simulink model "adarbha_hw6_mdl"  (Simulink 7.7)
settings: Solver=ode1  StartTime=0.0  StopTime=max(time_s)  FixedStep=0.00001  RelTol=1e-5
InitFcn:
  | adarbha_hw6
values from neighbouring files (symbols this model uses):
  Area = 2.7    [adarbha_hw6.m]    (also in hw6.m; hw6_code.m)
  Cd = 0.44    [adarbha_hw6.m]    (also in hw6.m; hw6_code.m)
  density = 1.224    [adarbha_hw6.m]    (also in hw6.m; hw6_code.m)
  Q = 20    [adarbha_hw6.m]    (also in hw6_code.m)
  R_batt = 0.1    [adarbha_hw6.m]    (also in hw6_code.m)
  radius_wheel_m = 0.41    [adarbha_hw6.m]    (also in hw6.m; hw6_code.m)
  rpm = 1:5000    [adarbha_hw6.m]    (also in hw6.m; hw6_code.m)
  Time = xlsread('Malibu_20100929_highway_Baseline','A:A')    [adarbha_hw6.m]    (also in hw6.m; hw6_code.m)
  time_s = time_scale*100    [adarbha_hw6.m]    (also in hw6.m; hw6_code.m)
  V_o = 300    [adarbha_hw6.m]    (also in hw6_code.m)
  vel_m_s = M_number*3    [adarbha_hw6.m]    (also in hw6.m; hw6_code.m)
  Velocity_kph = xlsread('Malibu_20100929_highway_Baseline','B:B')    [adarbha_hw6.m]    (also in hw6.m; hw6_code.m)
  weight_N = 16000    [adarbha_hw6.m]    (also in hw6.m; hw6_code.m)
undefined symbols (not defined in the file or in its folder): torque
libraries: simulink x1
settings Model: Creator=Arjun  LastModifiedBy=Arjun
settings DataIOCC: SignalLogging=off

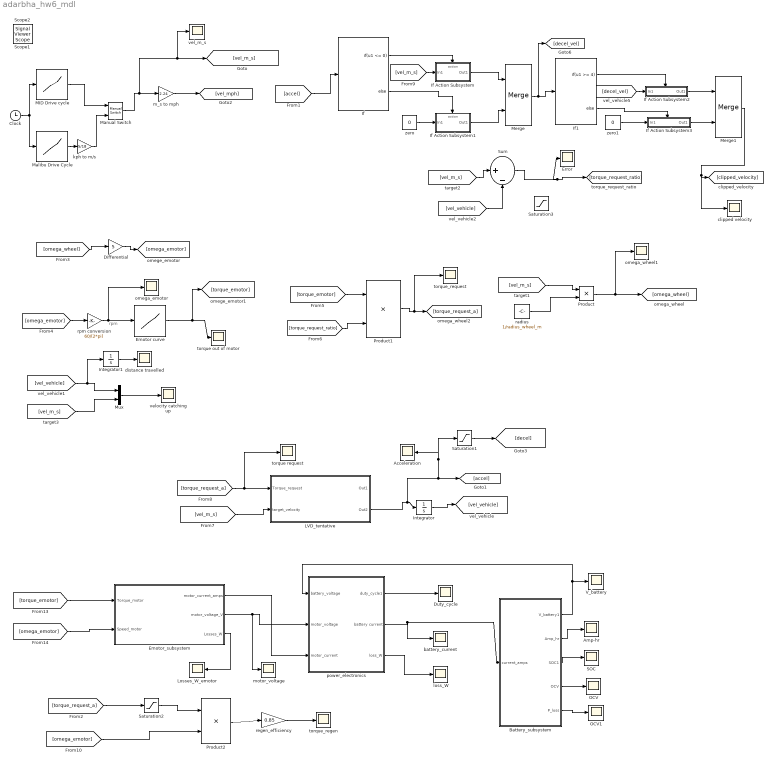
== system adarbha_hw6_mdl ==
  note: rpm
  Acceleration : Scope
      settings: SaveName=ScopeData11
  Amp-hr : Scope
      settings: SaveName=ScopeData23
  Battery_subsystem : Subsystem
      settings: MinAlgLoopOccurrences=on
  Clock : Clock
      settings: Decimation=10
  Differential : Gain  Gain=5
  Duty_cycle : Scope
      settings: SaveName=ScopeData22
  Emotor curve : Lookup_n-D  NumberOfTableDimensions=1  BreakpointsForDimension1=rpm  Table=torque  RndMeth=Simplest  InputSameDT=on
  Emotor_subsystem : Subsystem
  Error : Scope
      settings: SaveName=ScopeData17
  If : If  IfExpression=u1 <= 0
  If Action Subsystem : Subsystem  TreatAsAtomicUnit=on
  If Action Subsystem1 : Subsystem  TreatAsAtomicUnit=on
  If Action Subsystem2 : Subsystem  TreatAsAtomicUnit=on
  If Action Subsystem3 : Subsystem  TreatAsAtomicUnit=on
  If1 : If  IfExpression=u1 >= 4
  Integrator : Integrator
  Integrator1 : Integrator
  LVD_tentative : Subsystem
  Losses_W_emotor : Scope
      settings: SaveName=ScopeData19
  MID Drive cycle : Lookup_n-D  NumberOfTableDimensions=1  BreakpointsForDimension1=time_s  Table=vel_m_s  RndMeth=Simplest  InputSameDT=on
  Malibu Drive Cycle : Lookup_n-D  NumberOfTableDimensions=1  BreakpointsForDimension1=Time  Table=Velocity_kph  RndMeth=Simplest  InputSameDT=on
  Manual Switch : simulink/Signal Routing/Manual Switch  SystemSampleTime=-1  sw=1  action=0  varsize=off
  Merge : Merge
  Merge1 : Merge
  Mux : Mux  Inputs=2
  OCV : Scope
      settings: SaveName=ScopeData31
  OCV1 : Scope
      settings: SaveName=ScopeData33
  Product : Product  RndMeth=Zero
  Product1 : Product  RndMeth=Zero
  Product2 : Product  RndMeth=Zero
  SOC : Scope
      settings: SaveName=ScopeData28
  Saturation1 : Saturate  UpperLimit=0  LowerLimit=-100
  Saturation2 : Saturate  UpperLimit=0  LowerLimit=-Inf
  Saturation3 : Saturate  UpperLimit=1  LowerLimit=-1  ZeroCross=off
  Sum : Sum  Inputs=|+-
  V_battery : Scope
      settings: SaveName=ScopeData29
  battery_current : Scope
      settings: SaveName=ScopeData24
  clipped velocity : Scope
  distance travelled : Scope
      settings: SaveName=ScopeData25
  kph to m/s : Gain  Gain=5/18
  loss_W : Scope
      settings: SaveName=ScopeData20
  m_s to mph : Gain  Gain=2.24
  motor_voltage : Scope
      settings: SaveName=ScopeData26
  omega_emotor : Scope
      settings: SaveName=ScopeData7
  omega_wheel1 : Scope
      settings: SaveName=ScopeData4
  power_electronics : Subsystem
      settings: MinAlgLoopOccurrences=on
  radius : Constant  Value=1/radius_wheel_m
  regen_efficiency : Gain  Gain=0.85
  rpm conversion : Gain  Gain=60/(2*pi)
  torque out of motor : Scope
      settings: SaveName=ScopeData8
  torque request : Scope
      settings: SaveName=ScopeData12
  torque_regen : Scope
      settings: SaveName=ScopeData16
  torque_request : Scope
      settings: SaveName=ScopeData6
  vel_m_s : Scope
      settings: SaveName=ScopeData21
  velocity catching up : Scope
      settings: TimeRange=765.8724058416602  YMin=-1e+049  YMax=9.000000000000001e+049  SaveName=ScopeData18
  zero : Constant  Value=0
  zero1 : Constant  Value=0
  Scope1 : SignalViewerScope  IOType=viewer  NumInputPorts=5  RefreshTime=0.035000
  Scope2 : SignalViewerScope  IOType=viewer  RefreshTime=0.035000
  wires:
  m_s to mph/1 -> [vel_mph]
  Clock/1 -> MID Drive cycle/1, Malibu Drive Cycle/1
  [vel_m_s] -> Product/1
  Product/1 -> [omega_wheel], omega_wheel1/1
  radius/1 -> Product/2
  [torque_emotor] -> Product1/1
  [torque_request_ratio] -> Product1/2
  Product1/1 -> [torque_request_a], torque_request/1
  [omega_wheel] -> Differential/1
  Differential/1 -> [omega_emotor]
  [omega_emotor] -> rpm conversion/1
  rpm conversion/1 -> Emotor curve/1, omega_emotor/1
  Emotor curve/1 -> torque out of motor/1, [torque_emotor]
  [vel_m_s] -> LVD_tentative/2(target_velocity)
  [torque_request_a] -> LVD_tentative/1(Torque_request), torque request/1
  Integrator/1 -> [vel_vehicle]
  LVD_tentative/2(Out2) -> Integrator/1, [accel], Saturation1/1, Acceleration/1
  [vel_m_s] -> Sum/1
  [vel_vehicle] -> Sum/2
  [vel_m_s] -> Mux/2
  [vel_vehicle] -> Mux/1, Integrator1/1
  Mux/1 -> velocity catching up/1
  Sum/1 -> [torque_request_ratio], Error/1
  Saturation1/1 -> [decel]
  [accel] -> If/1
  If/1 -> If Action Subsystem/Action
  [vel_m_s] -> If Action Subsystem/1(In1)
  If/2 -> If Action Subsystem1/Action
  zero/1 -> If Action Subsystem1/1(In1)
  If Action Subsystem/1(Out1) -> Merge/1
  If Action Subsystem1/1(Out1) -> Merge/2
  Merge/1 -> If1/1, [decel_vel]
  If1/1 -> If Action Subsystem2/Action
  If1/2 -> If Action Subsystem3/Action
  [decel_vel] -> If Action Subsystem2/1(In1)
  zero1/1 -> If Action Subsystem3/1(In1)
  If Action Subsystem2/1(Out1) -> Merge1/1
  If Action Subsystem3/1(Out1) -> Merge1/2
  Merge1/1 -> clipped velocity/1, [clipped_velocity]
  MID Drive cycle/1 -> Manual Switch/1
  Manual Switch/1 -> m_s to mph/1, [vel_m_s], vel_m_s/1
  Malibu Drive Cycle/1 -> kph to m/s/1
  kph to m/s/1 -> Manual Switch/2
  Integrator1/1 -> distance travelled/1
  [torque_emotor] -> Emotor_subsystem/1(Torque_motor)
  [omega_emotor] -> Emotor_subsystem/2(Speed_motor)
  Emotor_subsystem/2(motor_voltage_V) -> power_electronics/2(motor_voltage), motor_voltage/1
  Emotor_subsystem/1(motor_current_amps) -> power_electronics/3(motor_current)
  power_electronics/2(battery current) -> battery_current/1, Battery_subsystem/1(current_amps)
  Battery_subsystem/1(V_battery1) -> V_battery/1, power_electronics/1(battery_voltage)
  Battery_subsystem/3(SOC1) -> SOC/1
  [torque_request_a] -> Saturation2/1
  Saturation2/1 -> Product2/1
  [omega_emotor] -> Product2/2
  Product2/1 -> regen_efficiency/1
  regen_efficiency/1 -> torque_regen/1
  Emotor_subsystem/3(Losses_W) -> Losses_W_emotor/1
  power_electronics/3(loss_W) -> loss_W/1
  power_electronics/1(duty_cycle1) -> Duty_cycle/1
  Battery_subsystem/2(Amp_hr) -> Amp-hr/1
  Battery_subsystem/4(OCV) -> OCV/1
  Battery_subsystem/5(P_loss) -> OCV1/1

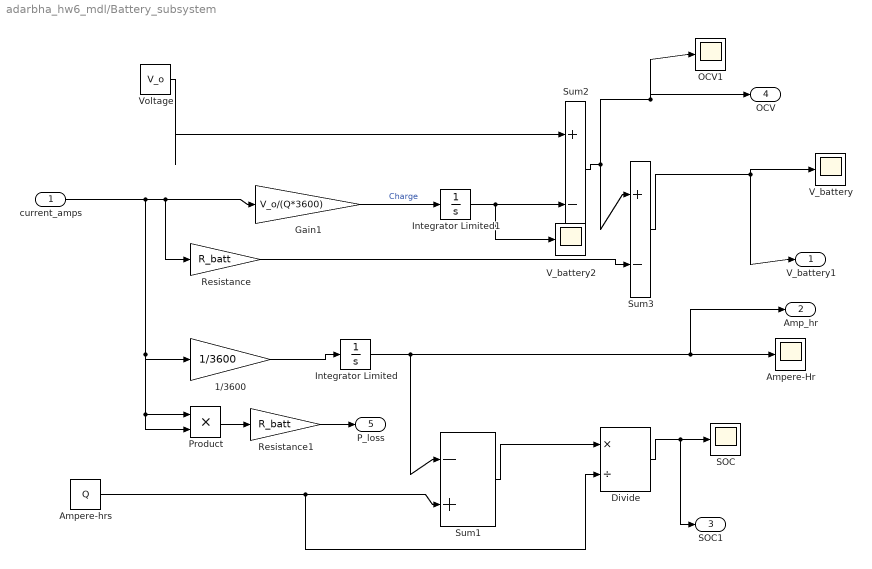
== system adarbha_hw6_mdl/Battery_subsystem ==
  current_amps : Inport
  1/3600 : Gain  Gain=1/3600
  Ampere-Hr : Scope
      settings: SaveName=ScopeData3
  Ampere-hrs : Constant  Value=Q
  Divide : Product  Inputs=*/
  Gain1 : Gain  Gain=V_o/(Q*3600)
  Integrator Limited : Integrator  LimitOutput=on  UpperSaturationLimit=Inf  LowerSaturationLimit=0
  Integrator Limited1 : Integrator  LimitOutput=on  UpperSaturationLimit=Inf  LowerSaturationLimit=0
  OCV1 : Scope
      settings: SaveName=ScopeData30
  Product : Product  RndMeth=Zero
  Resistance : Gain  Gain=R_batt
  Resistance1 : Gain  Gain=R_batt
  SOC : Scope
  Sum1 : Sum  Inputs=|-+
  Sum2 : Sum  Inputs=|+-
  Sum3 : Sum  Inputs=|+-
  V_battery : Scope
  V_battery2 : Scope
      settings: SaveName=ScopeData34
  Voltage : Constant  Value=V_o
  V_battery1 : Outport
  Amp_hr : Outport  Port=2
  SOC1 : Outport  Port=3
  OCV : Outport  Port=4
  P_loss : Outport  Port=5
  wires:
  Voltage/1 -> Sum2/1
  Gain1/1 -> Integrator Limited1/1  "Charge"
  Integrator Limited1/1 -> Sum2/2, V_battery2/1
  Resistance/1 -> Sum3/2
  Sum3/1 -> V_battery/1, V_battery1/1
  Ampere-hrs/1 -> Sum1/2, Divide/2
  Sum1/1 -> Divide/1
  Divide/1 -> SOC/1, SOC1/1
  Integrator Limited/1 -> Ampere-Hr/1, Amp_hr/1, Sum1/1
  1/3600/1 -> Integrator Limited/1
  Sum2/1 -> Sum3/1, OCV/1, OCV1/1
  current_amps/1 -> Gain1/1, Resistance/1, 1/3600/1, Product/1, Product/2
  Product/1 -> Resistance1/1
  Resistance1/1 -> P_loss/1

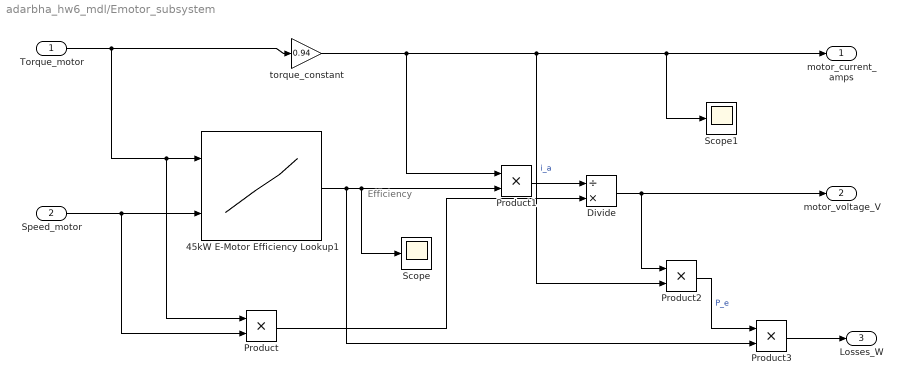
== system adarbha_hw6_mdl/Emotor_subsystem ==
  note: Efficiency
  Torque_motor : Inport
  Speed_motor : Inport  Port=2
  45kW E-Motor Efficiency Lookup1 : Lookup2D  RowIndex=[0,50,100,150,200,250,300,350,400,400,500,550]  ColumnIndex=[0,500,1000,1500,2000,2050,3000,3500,4000,4500]  Table=reshape([0.5,0.7,0.73,0.72,0.72,0.69,0.68,0.67,0.62,0.6,0.55,0.5,0.5,0.7,0.81,0.82,0.82,0.82,0.81,0.8,0.78,0.78,0.76,0.75,0.5,0.78,0.85,0.865,0.88,0.88,0.865,0.875,0.87,0.86,0.855,0.85,0.5,0.73,0.865,0.88,0.9,0.9,0.905,0.905,0.9,0.89,0.895,0.88,0.5,0.7,0.875,0.905,0.91,0.91,0.915,0.915,0.92,0.925,.925,0,0.5,0.8,0.875,0.905,0.915,0.92,0.92,0.925,0.93,0.93,0,0,0.5,0.76,0.875,0.9,0.925,0.94,0.95,0.96,0,0,0,0,0.5,0.76,0.875,0.9,0.925,0.935,0.935,0,0,0,0,0,0.5,0.75,0.87,0.905,0.925,0.925,0,0,0,0,0,0,0.5,0.75,0.865,0.905,0.92,0.92,0,0,0,0,0,0],12,10)
  Divide : Product  Inputs=/*
  Product{,1..3} (4 alike) : Product  RndMeth=Zero
  Scope : Scope
      settings: SaveName=ScopeData27
  Scope1 : Scope
      settings: SaveName=ScopeData32
  torque_constant : Gain  Gain=0.94
  motor_current_amps : Outport
  motor_voltage_V : Outport  Port=2
  Losses_W : Outport  Port=3
  wires:
  Torque_motor/1 -> torque_constant/1, 45kW E-Motor Efficiency Lookup1/1, Product/1
  Speed_motor/1 -> 45kW E-Motor Efficiency Lookup1/2, Product/2
  torque_constant/1 -> Product1/1, Product2/2, motor_current_amps/1, Scope1/1  "i_a"
  45kW E-Motor Efficiency Lookup1/1 -> Product3/2, Product1/2, Scope/1
  Product1/1 -> Divide/1
  Product/1 -> Divide/2
  Divide/1 -> motor_voltage_V/1, Product2/1
  Product2/1 -> Product3/1  "P_e"
  Product3/1 -> Losses_W/1

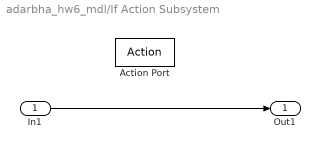
== system adarbha_hw6_mdl/If Action Subsystem ==
  In1 : Inport
  Action Port : ActionPort  ActionType=then
  Out1 : Outport
  wires:
  In1/1 -> Out1/1

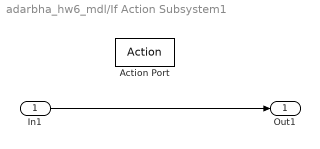
== system adarbha_hw6_mdl/If Action Subsystem1 ==
  In1 : Inport
  Action Port : ActionPort  ActionType=else
  Out1 : Outport
  wires:
  In1/1 -> Out1/1

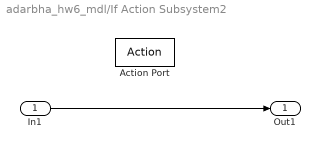
== system adarbha_hw6_mdl/If Action Subsystem2 ==
  In1 : Inport
  Action Port : ActionPort  ActionType=then
  Out1 : Outport
  wires:
  In1/1 -> Out1/1

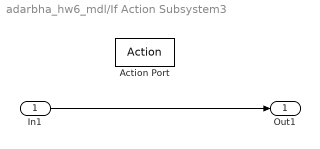
== system adarbha_hw6_mdl/If Action Subsystem3 ==
  In1 : Inport
  Action Port : ActionPort  ActionType=else
  Out1 : Outport
  wires:
  In1/1 -> Out1/1

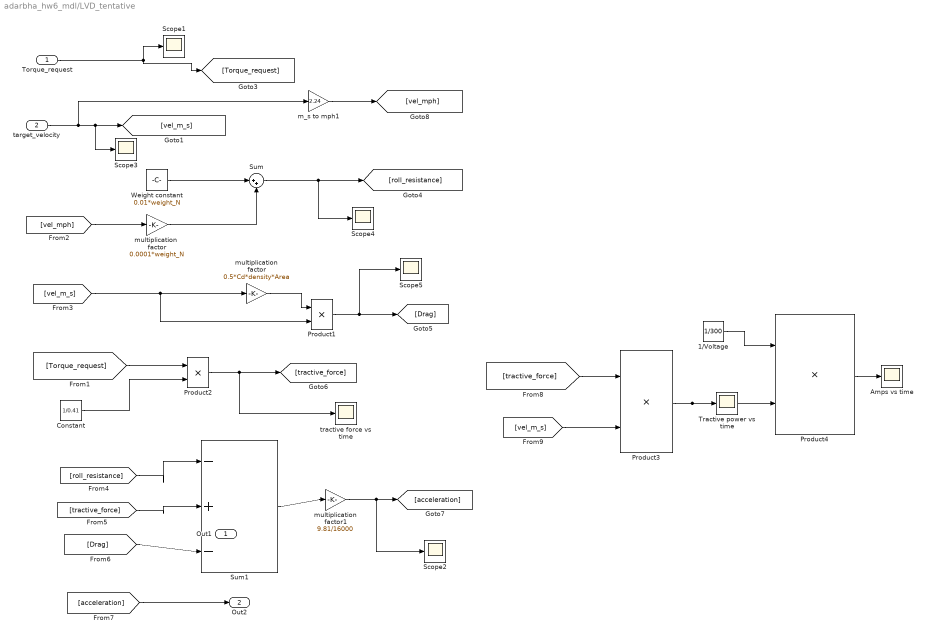
== system adarbha_hw6_mdl/LVD_tentative ==
  Torque_request : Inport
  target_velocity : Inport  Port=2
  1/Voltage : Constant  Value=1/300
  Amps vs time : Scope
      settings: SaveName=ScopeData15
  Constant : Constant  Value=1/0.41
  Product{1..4} (4 alike) : Product  RndMeth=Zero
  Scope{1..5} (5 alike) : Scope
      Scope1 settings: SaveName=ScopeData5
      Scope2 settings: SaveName=ScopeData6
      Scope3 settings: SaveName=ScopeData8
      Scope4 settings: SaveName=ScopeData9
      Scope5 settings: SaveName=ScopeData10
  Sum : Sum  Inputs=|++
  Sum1 : Sum  Inputs=|-+-
  Tractive power vs time : Scope
      settings: SaveName=ScopeData14
  Weight constant : Constant  Value=0.01*weight_N
  m_s to mph1 : Gain  Gain=2.24
  multiplication  factor : Gain  Gain=0.0001*weight_N
  multiplication factor : Gain  Gain=0.5*Cd*density*Area
  multiplication factor1 : Gain  Gain=9.81/16000
  tractive force vs time : Scope
      settings: SaveName=ScopeData13
  Out1 : Outport
  Out2 : Outport  Port=2
  wires:
  Weight constant/1 -> Sum/1
  multiplication  factor/1 -> Sum/2
  Sum/1 -> [roll_resistance], Scope4/1
  [vel_mph] -> multiplication  factor/1
  multiplication factor/1 -> Product1/1
  [vel_m_s] -> multiplication factor/1, Product1/2
  Product1/1 -> [Drag], Scope5/1
  [Torque_request] -> Product2/1
  Constant/1 -> Product2/2
  Product2/1 -> [tractive_force], tractive force vs time/1
  [roll_resistance] -> Sum1/1
  [tractive_force] -> Sum1/2
  [Drag] -> Sum1/3
  Sum1/1 -> multiplication factor1/1
  multiplication factor1/1 -> [acceleration], Scope2/1
  Torque_request/1 -> [Torque_request], Scope1/1
  target_velocity/1 -> m_s to mph1/1, [vel_m_s], Scope3/1
  m_s to mph1/1 -> [vel_mph]
  [acceleration] -> Out2/1
  [tractive_force] -> Product3/1
  [vel_m_s] -> Product3/2
  Product3/1 -> Tractive power vs time/1, Product4/2
  1/Voltage/1 -> Product4/1
  Product4/1 -> Amps vs time/1

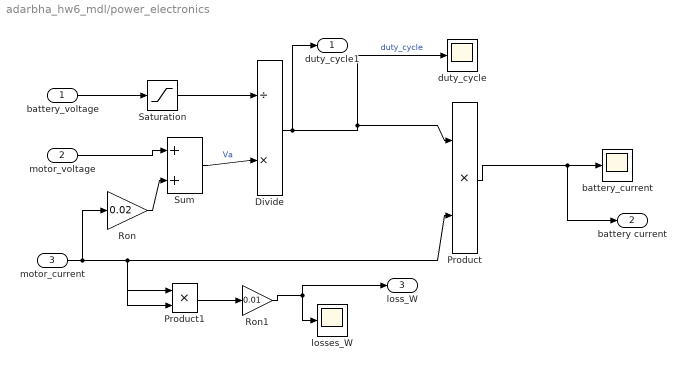
== system adarbha_hw6_mdl/power_electronics ==
  battery_voltage : Inport
  motor_voltage : Inport  Port=2
  motor_current : Inport  Port=3
  Divide : Product  Inputs=/*
  Product : Product  RndMeth=Zero
  Product1 : Product  RndMeth=Zero
  Ron : Gain  Gain=0.02
  Ron1 : Gain  Gain=0.01
  Saturation : Saturate  UpperLimit=1000000000000000  LowerLimit=0.1  ZeroCross=off
  Sum : Sum  Inputs=|++
  battery_current : Scope
  duty_cycle : Scope
  losses_W : Scope
      settings: SaveName=ScopeData2
  duty_cycle1 : Outport
  battery current : Outport  Port=2
  loss_W : Outport  Port=3
  wires:
  Saturation/1 -> Divide/1
  Sum/1 -> Divide/2  "Va"
  battery_voltage/1 -> Saturation/1
  motor_voltage/1 -> Sum/1
  motor_current/1 -> Ron/1, Product/2, Product1/1, Product1/2
  Divide/1 -> Product/1, duty_cycle/1, duty_cycle1/1  "duty_cycle"
  Product1/1 -> Ron1/1
  Product/1 -> battery_current/1, battery current/1
  Ron1/1 -> losses_W/1, loss_W/1
  Ron/1 -> Sum/2
